simulink model "ParetoBlending"  (R2017b)
settings: Solver=VariableStepAuto  StartTime=0.0  StopTime=20  RelTol=1e-3
undefined symbols (not defined in the file): Ts, Vx
libraries: simulink x2, mpclib x2, cstblocks x1
settings Model: Creator=The MathWorks, Inc.  LastModifiedBy=Yves
settings CodeAppCC: StateflowObjectComments=on
settings SimscapeCC: SimscapeNormalizeSystem=off

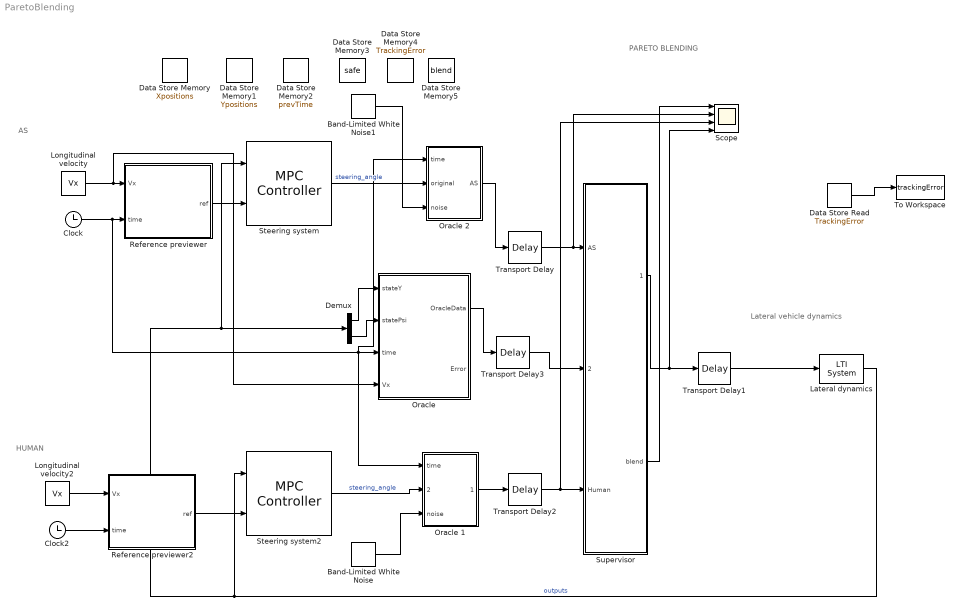
== system ParetoBlending ==
  note: PARETO BLENDING
  note: Lateral vehicle dynamics
  note: AS
  note: HUMAN
  Band-Limited White Noise : simulink/Sources/Band-Limited White Noise  Cov=[0]  Ts=1  seed=[23341]
  Band-Limited White Noise1 : simulink/Sources/Band-Limited White Noise  Cov=[0]  Ts=1  seed=[23341]
  Clock : Clock
  Clock2 : Clock
  Data Store Memory : DataStoreMemory  DataStoreName=Xpositions  ReadBeforeWriteMsg=warning  WriteAfterWriteMsg=warning  WriteAfterReadMsg=warning  ShowAdditionalParam=off  OutDataTypeStr=double  Dimensions=[1,5]
  Data Store Memory1 : DataStoreMemory  DataStoreName=Ypositions  ReadBeforeWriteMsg=warning  WriteAfterWriteMsg=warning  WriteAfterReadMsg=warning  ShowAdditionalParam=off  OutDataTypeStr=double  Dimensions=[1,5]
  Data Store Memory2 : DataStoreMemory  DataStoreName=prevTime  ReadBeforeWriteMsg=warning  WriteAfterWriteMsg=warning  WriteAfterReadMsg=warning  ShowAdditionalParam=off  OutDataTypeStr=double
  Data Store Memory3 : DataStoreMemory  DataStoreName=safe  ReadBeforeWriteMsg=warning  WriteAfterWriteMsg=warning  WriteAfterReadMsg=warning  ShowAdditionalParam=off  OutDataTypeStr=double
  Data Store Memory4 : DataStoreMemory  DataStoreName=TrackingError  ReadBeforeWriteMsg=warning  WriteAfterWriteMsg=warning  WriteAfterReadMsg=warning  ShowAdditionalParam=off  OutDataTypeStr=double
  Data Store Memory5 : DataStoreMemory  DataStoreName=blend  ReadBeforeWriteMsg=warning  WriteAfterWriteMsg=warning  WriteAfterReadMsg=warning  ShowAdditionalParam=off  OutDataTypeStr=double
  Data Store Read : DataStoreRead  DataStoreName=TrackingError  DataStoreElements=TrackingError
  Demux : Demux  Outputs=2
  Lateral dynamics : cstblocks/LTI System  sys=vehicle  IC=[]
  Longitudinal velocity : Constant  Value=Vx  SampleTime=Ts
  Longitudinal velocity2 : Constant  Value=Vx  SampleTime=Ts
  "Oracle " : MATLAB Function  TreatAsAtomicUnit=on  SystemSampleTime=0.1
  Oracle 1 : MATLAB Function  TreatAsAtomicUnit=on  SystemSampleTime=0.1
  Oracle 2 : MATLAB Function  TreatAsAtomicUnit=on  SystemSampleTime=0.1
  Reference previewer : MATLAB Function  TreatAsAtomicUnit=on  SystemSampleTime=Ts
  Reference previewer2 : MATLAB Function  TreatAsAtomicUnit=on  SystemSampleTime=Ts
  Scope : Scope  NumInputPorts=4
  Steering system : mpclib/MPC Controller  SCDEnableBlockLinearizationSpecification=on  mpcobj=ASMPC  is_multiple=0  enable_value=0  return_u0=off  ref_from_ws=off  ref_signal_name=[]  ref_preview=off  md_from_ws=off  md_signal_name=[]  md_preview=off  from_project=off  project_file=MPCtask.mat  md_inport=off  mv_inport=off  cost_outport=off  return_sequence=off  return_qpstatus=off  return_state=off  state_inport=off  lims_inport=off  cc_inport=off  ywt_inport=off  is_designfromscratch=0  uwt_inport=off  duwt_inport=off  rhoeps_inport=off  uref_inport=off  n_ts=0.1  n_p=10  n_mv=1  n_md=0  n_ud=0  n_mo=2  n_uo=0  BlockDataType=double  SampleTimeInherited=off  switch_inport=off
  Steering system2 : mpclib/MPC Controller  SCDEnableBlockLinearizationSpecification=on  mpcobj=HumanMPC  is_multiple=0  enable_value=0  return_u0=off  ref_from_ws=off  ref_signal_name=[]  ref_preview=off  md_from_ws=off  md_signal_name=[]  md_preview=off  from_project=off  project_file=MPCtask.mat  md_inport=off  mv_inport=off  cost_outport=off  return_sequence=off  return_qpstatus=off  return_state=off  state_inport=off  lims_inport=off  cc_inport=off  ywt_inport=off  is_designfromscratch=0  uwt_inport=off  duwt_inport=off  rhoeps_inport=off  uref_inport=off  n_ts=0.1  n_p=10  n_mv=1  n_md=0  n_ud=0  n_mo=2  n_uo=0  BlockDataType=double  SampleTimeInherited=off  switch_inport=off
  "Supervisor " : MATLAB Function  TreatAsAtomicUnit=on
  To Workspace : ToWorkspace  VariableName=trackingError  SaveFormat=Timeseries  SampleTime=-1
  Transport Delay : TransportDelay  DelayTime=0
  Transport Delay1 : TransportDelay  DelayTime=0.5
  Transport Delay2 : TransportDelay  DelayTime=0
  Transport Delay3 : TransportDelay  DelayTime=0
  wires:
  Longitudinal velocity/1 -> "Oracle "/4(Vx), Reference previewer/1(Vx)
  Clock/1 -> Oracle 2/1(time), Oracle 1/1(time), "Oracle "/3(time), Reference previewer/2(time)
  Reference previewer/1(ref) -> Steering system/2
  Lateral dynamics/1 -> Steering system2/1, Demux/1, Steering system/1  "outputs"
  "Supervisor "/1(blendedOutput) -> Scope/4, Transport Delay1/1
  Reference previewer2/1(ref) -> Steering system2/2
  Longitudinal velocity2/1 -> Reference previewer2/1(Vx)
  Clock2/1 -> Reference previewer2/2(time)
  "Oracle "/1(OracleData) -> Transport Delay3/1
  Demux/1 -> "Oracle "/1(stateY)
  Demux/2 -> "Oracle "/2(statePsi)
  Transport Delay/1 -> Scope/2, "Supervisor "/1(AS)
  Transport Delay1/1 -> Lateral dynamics/1
  Transport Delay2/1 -> "Supervisor "/3(Human), Scope/3
  Transport Delay3/1 -> "Supervisor "/2(OracleData)
  Band-Limited White Noise/1 -> Oracle 1/3(noise)
  Band-Limited White Noise1/1 -> Oracle 2/3(noise)
  Steering system/1 -> Oracle 2/2(original)  "steering_angle"
  Data Store Read/1 -> To Workspace/1
  "Supervisor "/2(blend) -> Scope/1
  Steering system2/1 -> Oracle 1/2(original)  "steering_angle"
  Oracle 1/1(Human) -> Transport Delay2/1
  Oracle 2/1(AS) -> Transport Delay/1

== matlab function ParetoBlending/Supervisor  ==
  data: AS input; blendedOutput output; OracleData input; Human input; blend output
function [blendedOutput, blend] = fcn(AS, OracleData, Human)


blend = OracleData;
blendedOutput = (AS*blend)+ ((1-blend)*Human);

%if(OracleData == 0)
 %   blendedOutput = 0;
%else
 %  blendedOutput = AS; 
end

== matlab function ParetoBlending/Reference previewer ==
  data: Vx input; time input; ref output
function ref = previewer(Vx,time)
% Get previewed reference trajectory

% Previw horizon is 10 sampling times (i.e. 10*0.1 = 1 seconds).
% Reference contains 2 signals (i.e. Y position and yaw angle).
ref = zeros(10,2); 

%% Previewing sequence
for ct = 1:10
   ref(ct,:) = doubleLaneChange(Vx,time + (ct-1)*0.1);
end

== matlab function ParetoBlending/Reference previewer2 ==
  data: Vx input; time input; ref output
function ref = previewer(Vx,time)
% Get previewed reference trajectory

% Previw horizon is 10 sampling times (i.e. 10*0.1 = 1 seconds).
% Reference contains 2 signals (i.e. Y position and yaw angle).
ref = zeros(10,2); 

%% Previewing sequence
for ct = 1:10
   ref(ct,:) = doubleLaneChange(Vx,time + (ct-1)*0.1);
end

== matlab function ParetoBlending/Oracle  ==
  settings: updateMethod=DISCRETE
  data: stateY input; statePsi input; OracleData output; Xpositions data_store_memory; Ypositions data_store_memory; prevTime data_store_memory; time input; Vx input; safe data_store_memory; Error output; TrackingError data_store_memory; blend data_store_memory
function [OracleData, Error] = fcn(stateY, statePsi, time, Vx)

obstacleX = [10,25,10,25,55,65,55,65,120,180,120,180];
obstacleY = [2,2,-1,-1,3,3,5,5,1,1,-4,-4];

global Xpositions ;
global prevTime;
global Ypositions ;
global safe; 
global TrackingError; 
global blend;

y = stateY;
psi = statePsi;

currentX = time * Vx;

collisionCourse = false;

if(prevTime+0.1 < time)
    
    prevTime = time;
    %get x and y position and add them to sliding window 
    
    Xpositions(1) = Xpositions(2);
    Xpositions(2) = Xpositions(3);
    Xpositions(3) = Xpositions(4);
    Xpositions(4) = Xpositions(5);
    Xpositions(5) = currentX;

    Ypositions(1) = Ypositions(2);
    Ypositions(2) = Ypositions(3);
    Ypositions(3) = Ypositions(4);
    Ypositions(4) = Ypositions(5);
    Ypositions(5) = y;
    
    p = polyfit(Xpositions,Ypositions,3);
    
    referencePath = zeros(3,2); 
    actualPath = zeros(3,2); 
    for ct = 1:3
       referencePath(ct,:) = doubleLaneChange(Vx,time + (ct-1)*0.1);
    end
    
    for ct2 = 1:3
       actualPath(ct2,:) = polyval(p, Vx*(time+(ct2-1)*0.1));
    end
    
    errorDif = abs(actualPath(1) - referencePath(1,1));
    isNotValid = isnan(errorDif);
    if(~isNotValid)
        blend = abs(actualPath(1) - referencePath(1,1));
        TrackingError = TrackingError + blend;
        disp(blend);
    end
    
     
    %check if on collision course
    %for index = 1:numel(obstacleX)
     %   obsX = obstacleX(index);
        %filter out obstacles within 5 meters
      %  if(obsX >= currentX && obsX <= currentX+5)
        %    disp('Obs in range');
         %   obsY = obstacleY(index);
         %   trajectoryForObs = polyval(p, obsX);
            
          %  disp(trajectoryForObs);
            %check if obstacle is within 0.5 meters of car
          %  if(abs(trajectoryForObs - obsY)<0.5)
           %     disp('Collosion course');
           %     collisionCourse = true;
           %    break;
           % end
      %  end
   % end
    
    
    %if(collisionCourse)
    %    blend = 0.5;
   % end
end

if(blend > 1)
    blend = 1;
end
%Safe = 0 , Unsafe = 1
OracleData = blend;
Error = TrackingError;
disp(TrackingError);

end

== matlab function ParetoBlending/Oracle 1 ==
  settings: updateMethod=DISCRETE
  data: time input; original input; noise input; Human output; Xpositions data_store_memory; Ypositions data_store_memory; prevTime data_store_memory; safe data_store_memory; TrackingError data_store_memory
function Human = fcn(time, original, noise)

if(time > 3 && time < 4)
    Human = original + noise;
else
    Human = original;

end

end

== matlab function ParetoBlending/Oracle 2 ==
  settings: updateMethod=DISCRETE
  data: time input; original input; noise input; AS output; Xpositions data_store_memory; Ypositions data_store_memory; prevTime data_store_memory; safe data_store_memory; TrackingError data_store_memory
function AS = fcn(time, original, noise)

if(time > 3 && time < 4)
    AS = original + noise;
else
    AS = original;

end

end
